simulink model "sistema_simples"  (R2018a)
settings: Solver=VariableStepAuto  StartTime=0.0  StopTime=10.0  RelTol=1e-3
values from neighbouring files (symbols this model uses):
  K = 0.169022678510371    (= 0.16902267851)    [entrada_arbitraria.m]    (also in entrada_arbitrária.m; teste_aleatorio_input.m; teste_bw.m = 1; teste_sinal_de_controle.m = 1)
  Td = 0.091354695916176    (= 0.0913546959162)    [entrada_arbitraria.m]    (also in entrada_arbitrária.m; parametros_pid.m = 1; teste_aleatorio_input.m; tsc.m = coef(3))
  Ti = 0.072109163345392    (= 0.0721091633454)    [entrada_arbitraria.m]    (also in entrada_arbitrária.m; parametros_pid.m = 1; teste_aleatorio_input.m; tsc.m = coef(2))
  wn = 8.036118730219977    (= 8.03611873022)    [entrada_arbitraria.m]    (also in entrada_arbitrária.m; parametros_pid.m; teste_aleatorio_input.m; teste_bw.m = 1)
  zeta = 0.900733958553509    (= 0.900733958554)    [entrada_arbitraria.m]    (also in entrada_arbitrária.m; parametros_pid.m; teste_aleatorio_input.m; teste_bw.m = 1)
libraries: cstblocks x2, simulink x1
settings Model: Creator=Eric Moretti  LastModifiedBy=Eric Moretti

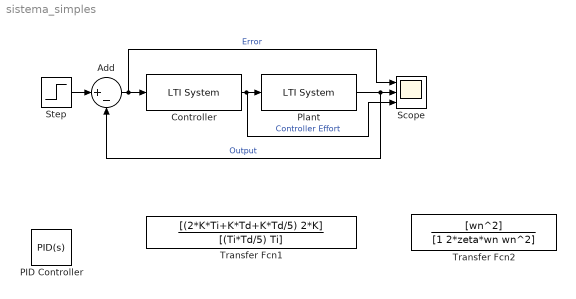
== system sistema_simples ==
  Add : Sum  Inputs=|+-
  Controller : cstblocks/LTI System  sys=P  IC=[]
  PID Controller : simulink/Continuous/PID Controller  Controller=PID  TimeDomain=Continuous-time  SampleTime=-1  IntegratorMethod=Forward Euler  FilterMethod=Forward Euler  Form=Parallel  UseFilter=on  ControllerParametersSource=internal  P=1  I=1  D=0  N=100  InitialConditionSource=internal  InitialConditionForIntegrator=0  InitialConditionForFilter=0  ExternalReset=none  LimitOutput=off  UpperSaturationLimit=inf  LowerSaturationLimit=-inf  LinearizeAsGain=on  AntiWindupMode=none  Kb=1  TrackingMode=off  Kt=1  PParamMin=[]  PParamMax=[]  IParamMin=[]  IParamMax=[]  DParamMin=[]  DParamMax=[]  NParamMin=[]  NParamMax=[]  KbParamMin=[]  KbParamMax=[]  KtParamMin=[]  KtParamMax=[]  POutMin=[]  POutMax=[]  IOutMin=[]  IOutMax=[]  DOutMin=[]  DOutMax=[]  NOutMin=[]  NOutMax=[]  KbOutMin=[]  KbOutMax=[]  KtOutMin=[]  KtOutMax=[]  IntegratorOutMin=[]  IntegratorOutMax=[]  FilterOutMin=[]  FilterOutMax=[]  SumOutMin=[]  SumOutMax=[]  SumI1OutMin=[]  SumI1OutMax=[]  SumI2OutMin=[]  SumI2OutMax=[]  SumI3OutMin=[]  SumI3OutMax=[]  SumDOutMin=[]  SumDOutMax=[]  SaturationOutMin=[]  SaturationOutMax=[]  IntegratorContinuousStateAttributes=''  IntegratorStateMustResolveToSignalObject=off  IntegratorRTWStateStorageClass=Auto  FilterContinuousStateAttributes=''  FilterStateMustResolveToSignalObject=off  FilterRTWStateStorageClass=Auto  DifferentiatorICPrevScaledInput=0  DifferentiatorOutMin=[]  DifferentiatorOutMax=[]  FilterDiffOutCoefMin=[]  FilterDiffOutCoefMax=[]  SumDenOutMin=[]  SumDenOutMax=[]  SumNumOutMin=[]  SumNumOutMax=[]  ReciprocalOutMin=[]  ReciprocalOutMax=[]  DivideOutMin=[]  DivideOutMax=[]  TunerSelectOption=Transfer Function Based (PID Tuner App)
  Plant : cstblocks/LTI System  sys=M  IC=[]
  Scope : Scope  NumInputPorts=3
  Step : Step  Time=0  SampleTime=0
  Transfer Fcn1 : TransferFcn  Numerator=[(2*K*Ti+K*Td+K*Td/5) 2*K]  Denominator=[(Ti*Td/5) Ti]
  Transfer Fcn2 : TransferFcn  Numerator=[wn^2]  Denominator=[1 2*zeta*wn wn^2]
  wires:
  Plant/1 -> Scope/2, Add/2  "Output"
  Add/1 -> Controller/1, Scope/1  "Error"
  Step/1 -> Add/1
  Controller/1 -> Scope/3, Plant/1  "Controller Effort"
